simulink model "SanazMotie"  (R2021a)
settings: Solver=VariableStepAuto  StartTime=0.0  StopTime=200  RelTol=1e-3
libraries: pid_lib x7
settings Model: Creator=Sanaz  LastModifiedBy=Sanaz

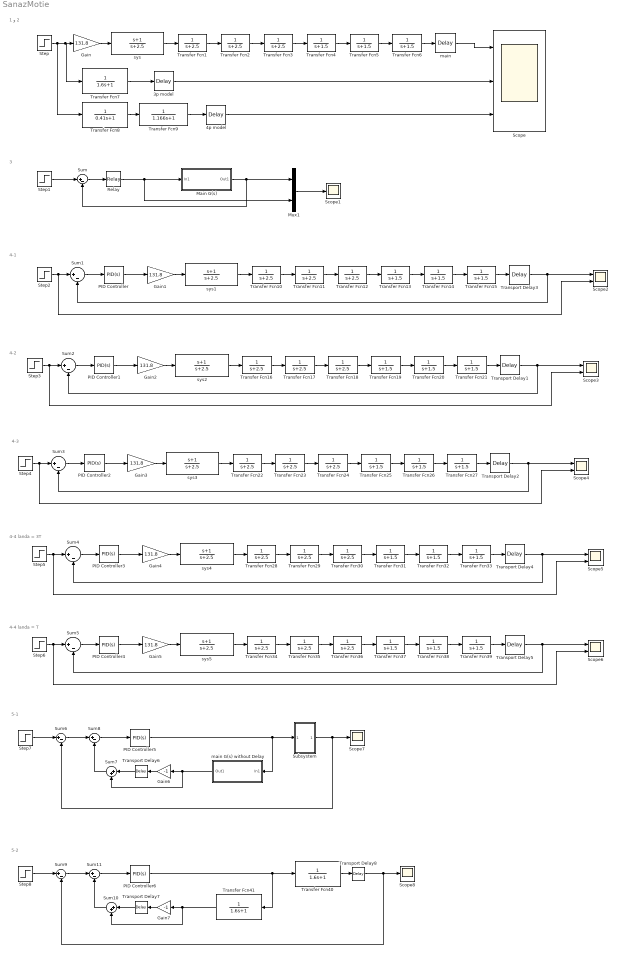
== system SanazMotie ==
  note: 5-1
  note: 3
  note: 4-1
  note: 1 و 2
  note: 4-2
  note: 4-3
  note: 4-4 landa = 3T
  note: 4-4 landa = T
  note: 5-2
  3p model : TransportDelay  DelayTime=3.7
  4p model : TransportDelay  DelayTime=3.7
  Gain{,1..5} (6 alike) : Gain  Gain=131.8
  Gain6 : Gain  Gain=-1
  Gain7 : Gain  Gain=-1
  Main G(s) : Subsystem
  Mux1 : Mux  Inputs=2
  PID Controller : pid_lib/PID Controller  Controller=PID  Form=Parallel  TimeDomain=Continuous-time  UseExternalTs=off  SampleTime=-1  IntegratorMethod=Forward Euler  FilterMethod=Forward Euler  ControllerParametersSource=internal  P=0.4  I=0.1  D=0  UseFilter=on  N=10  TunerSelectOption=Transfer Function Based (PID Tuner App)  InitialConditionSource=internal  InitialConditionForIntegrator=0  InitialConditionForFilter=0  DifferentiatorICPrevScaledInput=0  ExternalReset=none  TrackingMode=off  Kt=1  LimitOutput=off  SatLimitsSource=internal  UpperSaturationLimit=inf  LowerSaturationLimit=-inf  LinearizeAsGain=on  AntiWindupMode=none  Kb=1  POutMin=[]  POutMax=[]  IOutMin=[]  IOutMax=[]  DOutMin=[]  DOutMax=[]  NOutMin=[]  NOutMax=[]  SumOutMin=[]  SumOutMax=[]  SaturationOutMin=[]  SaturationOutMax=[]  PParamMin=[]  PParamMax=[]  IParamMin=[]  IParamMax=[]  DParamMin=[]  DParamMax=[]  NParamMin=[]  NParamMax=[]  KbParamMin=[]  KbParamMax=[]  KtParamMin=[]  KtParamMax=[]  KbOutMin=[]  KbOutMax=[]  KtOutMin=[]  KtOutMax=[]  IntegratorOutMin=[]  IntegratorOutMax=[]  FilterOutMin=[]  FilterOutMax=[]  SumI1OutMin=[]  SumI1OutMax=[]  SumI2OutMin=[]  SumI2OutMax=[]  SumI3OutMin=[]  SumI3OutMax=[]  SumI4OutMin=[]  SumI4OutMax=[]  SumDOutMin=[]  SumDOutMax=[]  DifferentiatorOutMin=[]  DifferentiatorOutMax=[]  FilterDiffOutCoefMin=[]  FilterDiffOutCoefMax=[]  ReciprocalOutMin=[]  ReciprocalOutMax=[]  SumDenOutMin=[]  SumDenOutMax=[]  SumNumOutMin=[]  SumNumOutMax=[]  DivideOutMin=[]  DivideOutMax=[]  UdiffTsProdOutMin=[]  UdiffTsProdOutMax=[]  NTsProdOutMin=[]  NTsProdOutMax=[]  UintegralTsProdOutMin=[]  UintegralTsProdOutMax=[]  UngainTsProdOutMin=[]  UngainTsProdOutMax=[]  IntegratorContinuousStateAttributes=''  IntegratorStateMustResolveToSignalObject=off  IntegratorRTWStateStorageClass=Auto  FilterContinuousStateAttributes=''  FilterStateMustResolveToSignalObject=off  FilterRTWStateStorageClass=Auto  ParallelPVariant=InternalParameters  IdealPVariant=Disabled  IVariant=InternalParameters  DVariant=InternalParameters  IntegratorVariant=Continuous  SatVariant=Disabled  AWVariant=Passthrough  PCopyVariant=Disabled  TRVariant=Disabled  FdbkBlocksVariant=Forward  IdealPFdbkVariant=Disabled  SatFdbkVariant=Disabled  DerivativeFilterVariant=ContFilter  NVariant=InternalParameters  NCopyVariant=Disabled  FilterICVariant=InternalICsFilter  IntegratorICVariant=InternalICs  ExternalResetVariant=Disabled  TRSumVariant=Passthrough  SumFdbkVariant=Disabled  SumVariant=Sum_PID  TsampFilterVariant=InternalTs  TsampNgainVariant=Passthrough  TsampIntegralVariant=Passthrough  ExternalSaturationOutDataTypeStr=Inherit: Same as second input
  PID Controller1 : pid_lib/PID Controller  Controller=PID  Form=Parallel  TimeDomain=Continuous-time  UseExternalTs=off  SampleTime=-1  IntegratorMethod=Forward Euler  FilterMethod=Forward Euler  ControllerParametersSource=internal  P=0.379787801338513  I=0.153670291898543  D=-0.495653562725149  UseFilter=on  N=0.201497063469897  TunerSelectOption=Transfer Function Based (PID Tuner App)  InitialConditionSource=internal  InitialConditionForIntegrator=0  InitialConditionForFilter=0  DifferentiatorICPrevScaledInput=0  ExternalReset=none  TrackingMode=off  Kt=1  LimitOutput=off  SatLimitsSource=internal  UpperSaturationLimit=inf  LowerSaturationLimit=-inf  LinearizeAsGain=on  AntiWindupMode=none  Kb=1  POutMin=[]  POutMax=[]  IOutMin=[]  IOutMax=[]  DOutMin=[]  DOutMax=[]  NOutMin=[]  NOutMax=[]  SumOutMin=[]  SumOutMax=[]  SaturationOutMin=[]  SaturationOutMax=[]  PParamMin=[]  PParamMax=[]  IParamMin=[]  IParamMax=[]  DParamMin=[]  DParamMax=[]  NParamMin=[]  NParamMax=[]  KbParamMin=[]  KbParamMax=[]  KtParamMin=[]  KtParamMax=[]  KbOutMin=[]  KbOutMax=[]  KtOutMin=[]  KtOutMax=[]  IntegratorOutMin=[]  IntegratorOutMax=[]  FilterOutMin=[]  FilterOutMax=[]  SumI1OutMin=[]  SumI1OutMax=[]  SumI2OutMin=[]  SumI2OutMax=[]  SumI3OutMin=[]  SumI3OutMax=[]  SumI4OutMin=[]  SumI4OutMax=[]  SumDOutMin=[]  SumDOutMax=[]  DifferentiatorOutMin=[]  DifferentiatorOutMax=[]  FilterDiffOutCoefMin=[]  FilterDiffOutCoefMax=[]  ReciprocalOutMin=[]  ReciprocalOutMax=[]  SumDenOutMin=[]  SumDenOutMax=[]  SumNumOutMin=[]  SumNumOutMax=[]  DivideOutMin=[]  DivideOutMax=[]  UdiffTsProdOutMin=[]  UdiffTsProdOutMax=[]  NTsProdOutMin=[]  NTsProdOutMax=[]  UintegralTsProdOutMin=[]  UintegralTsProdOutMax=[]  UngainTsProdOutMin=[]  UngainTsProdOutMax=[]  IntegratorContinuousStateAttributes=''  IntegratorStateMustResolveToSignalObject=off  IntegratorRTWStateStorageClass=Auto  FilterContinuousStateAttributes=''  FilterStateMustResolveToSignalObject=off  FilterRTWStateStorageClass=Auto  ParallelPVariant=InternalParameters  IdealPVariant=Disabled  IVariant=InternalParameters  DVariant=InternalParameters  IntegratorVariant=Continuous  SatVariant=Disabled  AWVariant=Passthrough  PCopyVariant=Disabled  TRVariant=Disabled  FdbkBlocksVariant=Forward  IdealPFdbkVariant=Disabled  SatFdbkVariant=Disabled  DerivativeFilterVariant=ContFilter  NVariant=InternalParameters  NCopyVariant=Disabled  FilterICVariant=InternalICsFilter  IntegratorICVariant=InternalICs  ExternalResetVariant=Disabled  TRSumVariant=Passthrough  SumFdbkVariant=Disabled  SumVariant=Sum_PID  TsampFilterVariant=InternalTs  TsampNgainVariant=Passthrough  TsampIntegralVariant=Passthrough  ExternalSaturationOutDataTypeStr=Inherit: Same as second input
  PID Controller2 : pid_lib/PID Controller  Controller=PID  Form=Parallel  TimeDomain=Continuous-time  UseExternalTs=off  SampleTime=-1  IntegratorMethod=Forward Euler  FilterMethod=Forward Euler  ControllerParametersSource=internal  P=0.258  I=0.02  D=0.6  UseFilter=on  N=3  TunerSelectOption=Frequency Response Based  InitialConditionSource=internal  InitialConditionForIntegrator=0  InitialConditionForFilter=0  DifferentiatorICPrevScaledInput=0  ExternalReset=none  TrackingMode=off  Kt=1  LimitOutput=off  SatLimitsSource=internal  UpperSaturationLimit=inf  LowerSaturationLimit=-inf  LinearizeAsGain=on  AntiWindupMode=none  Kb=1  POutMin=[]  POutMax=[]  IOutMin=[]  IOutMax=[]  DOutMin=[]  DOutMax=[]  NOutMin=[]  NOutMax=[]  SumOutMin=[]  SumOutMax=[]  SaturationOutMin=[]  SaturationOutMax=[]  PParamMin=[]  PParamMax=[]  IParamMin=[]  IParamMax=[]  DParamMin=[]  DParamMax=[]  NParamMin=[]  NParamMax=[]  KbParamMin=[]  KbParamMax=[]  KtParamMin=[]  KtParamMax=[]  KbOutMin=[]  KbOutMax=[]  KtOutMin=[]  KtOutMax=[]  IntegratorOutMin=[]  IntegratorOutMax=[]  FilterOutMin=[]  FilterOutMax=[]  SumI1OutMin=[]  SumI1OutMax=[]  SumI2OutMin=[]  SumI2OutMax=[]  SumI3OutMin=[]  SumI3OutMax=[]  SumI4OutMin=[]  SumI4OutMax=[]  SumDOutMin=[]  SumDOutMax=[]  DifferentiatorOutMin=[]  DifferentiatorOutMax=[]  FilterDiffOutCoefMin=[]  FilterDiffOutCoefMax=[]  ReciprocalOutMin=[]  ReciprocalOutMax=[]  SumDenOutMin=[]  SumDenOutMax=[]  SumNumOutMin=[]  SumNumOutMax=[]  DivideOutMin=[]  DivideOutMax=[]  UdiffTsProdOutMin=[]  UdiffTsProdOutMax=[]  NTsProdOutMin=[]  NTsProdOutMax=[]  UintegralTsProdOutMin=[]  UintegralTsProdOutMax=[]  UngainTsProdOutMin=[]  UngainTsProdOutMax=[]  IntegratorContinuousStateAttributes=''  IntegratorStateMustResolveToSignalObject=off  IntegratorRTWStateStorageClass=Auto  FilterContinuousStateAttributes=''  FilterStateMustResolveToSignalObject=off  FilterRTWStateStorageClass=Auto  ParallelPVariant=InternalParameters  IdealPVariant=Disabled  IVariant=InternalParameters  DVariant=InternalParameters  IntegratorVariant=Continuous  SatVariant=Disabled  AWVariant=Passthrough  PCopyVariant=Disabled  TRVariant=Disabled  FdbkBlocksVariant=Forward  IdealPFdbkVariant=Disabled  SatFdbkVariant=Disabled  DerivativeFilterVariant=ContFilter  NVariant=InternalParameters  NCopyVariant=Disabled  FilterICVariant=InternalICsFilter  IntegratorICVariant=InternalICs  ExternalResetVariant=Disabled  TRSumVariant=Passthrough  SumFdbkVariant=Disabled  SumVariant=Sum_PID  TsampFilterVariant=InternalTs  TsampNgainVariant=Passthrough  TsampIntegralVariant=Passthrough  ExternalSaturationOutDataTypeStr=Inherit: Same as second input
  PID Controller3 : pid_lib/PID Controller  Controller=PID  Form=Parallel  TimeDomain=Continuous-time  UseExternalTs=off  SampleTime=-1  IntegratorMethod=Forward Euler  FilterMethod=Forward Euler  ControllerParametersSource=internal  P=0.517  I=0.15  D=0.44  UseFilter=on  N=3  TunerSelectOption=Frequency Response Based  InitialConditionSource=internal  InitialConditionForIntegrator=0  InitialConditionForFilter=0  DifferentiatorICPrevScaledInput=0  ExternalReset=none  TrackingMode=off  Kt=1  LimitOutput=off  SatLimitsSource=internal  UpperSaturationLimit=inf  LowerSaturationLimit=-inf  LinearizeAsGain=on  AntiWindupMode=none  Kb=1  POutMin=[]  POutMax=[]  IOutMin=[]  IOutMax=[]  DOutMin=[]  DOutMax=[]  NOutMin=[]  NOutMax=[]  SumOutMin=[]  SumOutMax=[]  SaturationOutMin=[]  SaturationOutMax=[]  PParamMin=[]  PParamMax=[]  IParamMin=[]  IParamMax=[]  DParamMin=[]  DParamMax=[]  NParamMin=[]  NParamMax=[]  KbParamMin=[]  KbParamMax=[]  KtParamMin=[]  KtParamMax=[]  KbOutMin=[]  KbOutMax=[]  KtOutMin=[]  KtOutMax=[]  IntegratorOutMin=[]  IntegratorOutMax=[]  FilterOutMin=[]  FilterOutMax=[]  SumI1OutMin=[]  SumI1OutMax=[]  SumI2OutMin=[]  SumI2OutMax=[]  SumI3OutMin=[]  SumI3OutMax=[]  SumI4OutMin=[]  SumI4OutMax=[]  SumDOutMin=[]  SumDOutMax=[]  DifferentiatorOutMin=[]  DifferentiatorOutMax=[]  FilterDiffOutCoefMin=[]  FilterDiffOutCoefMax=[]  ReciprocalOutMin=[]  ReciprocalOutMax=[]  SumDenOutMin=[]  SumDenOutMax=[]  SumNumOutMin=[]  SumNumOutMax=[]  DivideOutMin=[]  DivideOutMax=[]  UdiffTsProdOutMin=[]  UdiffTsProdOutMax=[]  NTsProdOutMin=[]  NTsProdOutMax=[]  UintegralTsProdOutMin=[]  UintegralTsProdOutMax=[]  UngainTsProdOutMin=[]  UngainTsProdOutMax=[]  IntegratorContinuousStateAttributes=''  IntegratorStateMustResolveToSignalObject=off  IntegratorRTWStateStorageClass=Auto  FilterContinuousStateAttributes=''  FilterStateMustResolveToSignalObject=off  FilterRTWStateStorageClass=Auto  ParallelPVariant=InternalParameters  IdealPVariant=Disabled  IVariant=InternalParameters  DVariant=InternalParameters  IntegratorVariant=Continuous  SatVariant=Disabled  AWVariant=Passthrough  PCopyVariant=Disabled  TRVariant=Disabled  FdbkBlocksVariant=Forward  IdealPFdbkVariant=Disabled  SatFdbkVariant=Disabled  DerivativeFilterVariant=ContFilter  NVariant=InternalParameters  NCopyVariant=Disabled  FilterICVariant=InternalICsFilter  IntegratorICVariant=InternalICs  ExternalResetVariant=Disabled  TRSumVariant=Passthrough  SumFdbkVariant=Disabled  SumVariant=Sum_PID  TsampFilterVariant=InternalTs  TsampNgainVariant=Passthrough  TsampIntegralVariant=Passthrough  ExternalSaturationOutDataTypeStr=Inherit: Same as second input
  PID Controller4 : pid_lib/PID Controller  Controller=PID  Form=Parallel  TimeDomain=Continuous-time  UseExternalTs=off  SampleTime=-1  IntegratorMethod=Forward Euler  FilterMethod=Forward Euler  ControllerParametersSource=internal  P=1.01  I=0.3  D=0.87  UseFilter=on  N=3  TunerSelectOption=Frequency Response Based  InitialConditionSource=internal  InitialConditionForIntegrator=0  InitialConditionForFilter=0  DifferentiatorICPrevScaledInput=0  ExternalReset=none  TrackingMode=off  Kt=1  LimitOutput=off  SatLimitsSource=internal  UpperSaturationLimit=inf  LowerSaturationLimit=-inf  LinearizeAsGain=on  AntiWindupMode=none  Kb=1  POutMin=[]  POutMax=[]  IOutMin=[]  IOutMax=[]  DOutMin=[]  DOutMax=[]  NOutMin=[]  NOutMax=[]  SumOutMin=[]  SumOutMax=[]  SaturationOutMin=[]  SaturationOutMax=[]  PParamMin=[]  PParamMax=[]  IParamMin=[]  IParamMax=[]  DParamMin=[]  DParamMax=[]  NParamMin=[]  NParamMax=[]  KbParamMin=[]  KbParamMax=[]  KtParamMin=[]  KtParamMax=[]  KbOutMin=[]  KbOutMax=[]  KtOutMin=[]  KtOutMax=[]  IntegratorOutMin=[]  IntegratorOutMax=[]  FilterOutMin=[]  FilterOutMax=[]  SumI1OutMin=[]  SumI1OutMax=[]  SumI2OutMin=[]  SumI2OutMax=[]  SumI3OutMin=[]  SumI3OutMax=[]  SumI4OutMin=[]  SumI4OutMax=[]  SumDOutMin=[]  SumDOutMax=[]  DifferentiatorOutMin=[]  DifferentiatorOutMax=[]  FilterDiffOutCoefMin=[]  FilterDiffOutCoefMax=[]  ReciprocalOutMin=[]  ReciprocalOutMax=[]  SumDenOutMin=[]  SumDenOutMax=[]  SumNumOutMin=[]  SumNumOutMax=[]  DivideOutMin=[]  DivideOutMax=[]  UdiffTsProdOutMin=[]  UdiffTsProdOutMax=[]  NTsProdOutMin=[]  NTsProdOutMax=[]  UintegralTsProdOutMin=[]  UintegralTsProdOutMax=[]  UngainTsProdOutMin=[]  UngainTsProdOutMax=[]  IntegratorContinuousStateAttributes=''  IntegratorStateMustResolveToSignalObject=off  IntegratorRTWStateStorageClass=Auto  FilterContinuousStateAttributes=''  FilterStateMustResolveToSignalObject=off  FilterRTWStateStorageClass=Auto  ParallelPVariant=InternalParameters  IdealPVariant=Disabled  IVariant=InternalParameters  DVariant=InternalParameters  IntegratorVariant=Continuous  SatVariant=Disabled  AWVariant=Passthrough  PCopyVariant=Disabled  TRVariant=Disabled  FdbkBlocksVariant=Forward  IdealPFdbkVariant=Disabled  SatFdbkVariant=Disabled  DerivativeFilterVariant=ContFilter  NVariant=InternalParameters  NCopyVariant=Disabled  FilterICVariant=InternalICsFilter  IntegratorICVariant=InternalICs  ExternalResetVariant=Disabled  TRSumVariant=Passthrough  SumFdbkVariant=Disabled  SumVariant=Sum_PID  TsampFilterVariant=InternalTs  TsampNgainVariant=Passthrough  TsampIntegralVariant=Passthrough  ExternalSaturationOutDataTypeStr=Inherit: Same as second input
  PID Controller5 : pid_lib/PID Controller  Controller=PID  Form=Parallel  TimeDomain=Continuous-time  UseExternalTs=off  SampleTime=-1  IntegratorMethod=Forward Euler  FilterMethod=Forward Euler  ControllerParametersSource=internal  P=0.38  I=0.15  D=-0.5  UseFilter=on  N=0.2  TunerSelectOption=Transfer Function Based (PID Tuner App)  InitialConditionSource=internal  InitialConditionForIntegrator=0  InitialConditionForFilter=0  DifferentiatorICPrevScaledInput=0  ExternalReset=none  TrackingMode=off  Kt=1  LimitOutput=off  SatLimitsSource=internal  UpperSaturationLimit=inf  LowerSaturationLimit=-inf  LinearizeAsGain=on  AntiWindupMode=none  Kb=1  POutMin=[]  POutMax=[]  IOutMin=[]  IOutMax=[]  DOutMin=[]  DOutMax=[]  NOutMin=[]  NOutMax=[]  SumOutMin=[]  SumOutMax=[]  SaturationOutMin=[]  SaturationOutMax=[]  PParamMin=[]  PParamMax=[]  IParamMin=[]  IParamMax=[]  DParamMin=[]  DParamMax=[]  NParamMin=[]  NParamMax=[]  KbParamMin=[]  KbParamMax=[]  KtParamMin=[]  KtParamMax=[]  KbOutMin=[]  KbOutMax=[]  KtOutMin=[]  KtOutMax=[]  IntegratorOutMin=[]  IntegratorOutMax=[]  FilterOutMin=[]  FilterOutMax=[]  SumI1OutMin=[]  SumI1OutMax=[]  SumI2OutMin=[]  SumI2OutMax=[]  SumI3OutMin=[]  SumI3OutMax=[]  SumI4OutMin=[]  SumI4OutMax=[]  SumDOutMin=[]  SumDOutMax=[]  DifferentiatorOutMin=[]  DifferentiatorOutMax=[]  FilterDiffOutCoefMin=[]  FilterDiffOutCoefMax=[]  ReciprocalOutMin=[]  ReciprocalOutMax=[]  SumDenOutMin=[]  SumDenOutMax=[]  SumNumOutMin=[]  SumNumOutMax=[]  DivideOutMin=[]  DivideOutMax=[]  UdiffTsProdOutMin=[]  UdiffTsProdOutMax=[]  NTsProdOutMin=[]  NTsProdOutMax=[]  UintegralTsProdOutMin=[]  UintegralTsProdOutMax=[]  UngainTsProdOutMin=[]  UngainTsProdOutMax=[]  IntegratorContinuousStateAttributes=''  IntegratorStateMustResolveToSignalObject=off  IntegratorRTWStateStorageClass=Auto  FilterContinuousStateAttributes=''  FilterStateMustResolveToSignalObject=off  FilterRTWStateStorageClass=Auto  ParallelPVariant=InternalParameters  IdealPVariant=Disabled  IVariant=InternalParameters  DVariant=InternalParameters  IntegratorVariant=Continuous  SatVariant=Disabled  AWVariant=Passthrough  PCopyVariant=Disabled  TRVariant=Disabled  FdbkBlocksVariant=Forward  IdealPFdbkVariant=Disabled  SatFdbkVariant=Disabled  DerivativeFilterVariant=ContFilter  NVariant=InternalParameters  NCopyVariant=Disabled  FilterICVariant=InternalICsFilter  IntegratorICVariant=InternalICs  ExternalResetVariant=Disabled  TRSumVariant=Passthrough  SumFdbkVariant=Disabled  SumVariant=Sum_PID  TsampFilterVariant=InternalTs  TsampNgainVariant=Passthrough  TsampIntegralVariant=Passthrough  ExternalSaturationOutDataTypeStr=Inherit: Same as second input
  PID Controller6 : pid_lib/PID Controller  Controller=PID  Form=Parallel  TimeDomain=Continuous-time  UseExternalTs=off  SampleTime=-1  IntegratorMethod=Forward Euler  FilterMethod=Forward Euler  ControllerParametersSource=internal  P=0.38  I=0.15  D=-0.5  UseFilter=on  N=0.2  TunerSelectOption=Transfer Function Based (PID Tuner App)  InitialConditionSource=internal  InitialConditionForIntegrator=0  InitialConditionForFilter=0  DifferentiatorICPrevScaledInput=0  ExternalReset=none  TrackingMode=off  Kt=1  LimitOutput=off  SatLimitsSource=internal  UpperSaturationLimit=inf  LowerSaturationLimit=-inf  LinearizeAsGain=on  AntiWindupMode=none  Kb=1  POutMin=[]  POutMax=[]  IOutMin=[]  IOutMax=[]  DOutMin=[]  DOutMax=[]  NOutMin=[]  NOutMax=[]  SumOutMin=[]  SumOutMax=[]  SaturationOutMin=[]  SaturationOutMax=[]  PParamMin=[]  PParamMax=[]  IParamMin=[]  IParamMax=[]  DParamMin=[]  DParamMax=[]  NParamMin=[]  NParamMax=[]  KbParamMin=[]  KbParamMax=[]  KtParamMin=[]  KtParamMax=[]  KbOutMin=[]  KbOutMax=[]  KtOutMin=[]  KtOutMax=[]  IntegratorOutMin=[]  IntegratorOutMax=[]  FilterOutMin=[]  FilterOutMax=[]  SumI1OutMin=[]  SumI1OutMax=[]  SumI2OutMin=[]  SumI2OutMax=[]  SumI3OutMin=[]  SumI3OutMax=[]  SumI4OutMin=[]  SumI4OutMax=[]  SumDOutMin=[]  SumDOutMax=[]  DifferentiatorOutMin=[]  DifferentiatorOutMax=[]  FilterDiffOutCoefMin=[]  FilterDiffOutCoefMax=[]  ReciprocalOutMin=[]  ReciprocalOutMax=[]  SumDenOutMin=[]  SumDenOutMax=[]  SumNumOutMin=[]  SumNumOutMax=[]  DivideOutMin=[]  DivideOutMax=[]  UdiffTsProdOutMin=[]  UdiffTsProdOutMax=[]  NTsProdOutMin=[]  NTsProdOutMax=[]  UintegralTsProdOutMin=[]  UintegralTsProdOutMax=[]  UngainTsProdOutMin=[]  UngainTsProdOutMax=[]  IntegratorContinuousStateAttributes=''  IntegratorStateMustResolveToSignalObject=off  IntegratorRTWStateStorageClass=Auto  FilterContinuousStateAttributes=''  FilterStateMustResolveToSignalObject=off  FilterRTWStateStorageClass=Auto  ParallelPVariant=InternalParameters  IdealPVariant=Disabled  IVariant=InternalParameters  DVariant=InternalParameters  IntegratorVariant=Continuous  SatVariant=Disabled  AWVariant=Passthrough  PCopyVariant=Disabled  TRVariant=Disabled  FdbkBlocksVariant=Forward  IdealPFdbkVariant=Disabled  SatFdbkVariant=Disabled  DerivativeFilterVariant=ContFilter  NVariant=InternalParameters  NCopyVariant=Disabled  FilterICVariant=InternalICsFilter  IntegratorICVariant=InternalICs  ExternalResetVariant=Disabled  TRSumVariant=Passthrough  SumFdbkVariant=Disabled  SumVariant=Sum_PID  TsampFilterVariant=InternalTs  TsampNgainVariant=Passthrough  TsampIntegralVariant=Passthrough  ExternalSaturationOutDataTypeStr=Inherit: Same as second input
  Relay : Relay  OnOutputValue=5  OffOutputValue=-5
  Scope : Scope  NumInputPorts=3
  Scope1 : Scope
  Scope{2..6} (5 alike) : Scope  NumInputPorts=2
  Scope7 : Scope
  Scope8 : Scope
  Step{,1,7..8} (4 alike) : Step  Time=0  SampleTime=0
  Step{2..6} (5 alike) : Step  SampleTime=0
  Subsystem : Subsystem
  Sum{,1..6,8..9,11} (10 alike) : Sum  Inputs=|+-
  Sum10 : Sum  Inputs=|++
  Sum7 : Sum  Inputs=|++
  Transfer Fcn{1..3,10..12,16..18,22..24,28..30,34..36} (18 alike) : TransferFcn  Denominator=[1 2.5]
  Transfer Fcn{4..6,13..15,19..21,25..27,31..33,37..39} (18 alike) : TransferFcn  Denominator=[1 1.5]
  Transfer Fcn40 : TransferFcn  Denominator=[1.6 1]
  Transfer Fcn41 : TransferFcn  Denominator=[1.6 1]
  Transfer Fcn7 : TransferFcn  Denominator=[1.6 1]
  Transfer Fcn8 : TransferFcn  Denominator=[0.41 1]
  Transfer Fcn9 : TransferFcn  Denominator=[1.166 1]
  Transport Delay{1..5} (5 alike) : TransportDelay  DelayTime=2.5
  Transport Delay6 : TransportDelay  DelayTime=3.7
  Transport Delay7 : TransportDelay  DelayTime=3.7
  Transport Delay8 : TransportDelay  DelayTime=3.7
  main : TransportDelay  DelayTime=2.5
  main G(s) without Delay : Subsystem
  sys{,1..5} (6 alike) : TransferFcn  Numerator=[1 1]  Denominator=[1 2.5]
  wires:
  main/1 -> Scope/1
  Step/1 -> Transfer Fcn8/1, Transfer Fcn7/1, Gain/1
  Transfer Fcn3/1 -> Transfer Fcn4/1
  Transfer Fcn5/1 -> Transfer Fcn6/1
  Transfer Fcn2/1 -> Transfer Fcn3/1
  Transfer Fcn4/1 -> Transfer Fcn5/1
  Transfer Fcn6/1 -> main/1
  sys/1 -> Transfer Fcn1/1
  Transfer Fcn1/1 -> Transfer Fcn2/1
  Transfer Fcn8/1 -> Transfer Fcn9/1
  Transfer Fcn7/1 -> 3p model/1
  Transfer Fcn9/1 -> 4p model/1
  Gain/1 -> sys/1
  Step1/1 -> Sum/1
  Mux1/1 -> Scope1/1
  Relay/1 -> Mux1/2, Main G(s)/1(In1)
  Main G(s)/1(Out1) -> Sum/2, Mux1/1
  Sum/1 -> Relay/1
  Gain1/1 -> sys1/1
  Transfer Fcn10/1 -> Transfer Fcn11/1
  Transfer Fcn14/1 -> Transfer Fcn15/1
  Transfer Fcn11/1 -> Transfer Fcn12/1
  Transfer Fcn15/1 -> Transport Delay3/1
  sys1/1 -> Transfer Fcn10/1
  Transfer Fcn13/1 -> Transfer Fcn14/1
  Transfer Fcn12/1 -> Transfer Fcn13/1
  PID Controller/1 -> Gain1/1
  Step2/1 -> Scope2/2, Sum1/1
  Sum1/1 -> PID Controller/1
  Transport Delay3/1 -> Sum1/2, Scope2/1
  3p model/1 -> Scope/2
  4p model/1 -> Scope/3
  Transfer Fcn20/1 -> Transfer Fcn21/1
  Transfer Fcn18/1 -> Transfer Fcn19/1
  Transfer Fcn19/1 -> Transfer Fcn20/1
  Step3/1 -> Scope3/2, Sum2/1
  sys2/1 -> Transfer Fcn16/1
  PID Controller1/1 -> Gain2/1
  Transfer Fcn16/1 -> Transfer Fcn17/1
  Sum2/1 -> PID Controller1/1
  Transport Delay1/1 -> Sum2/2, Scope3/1
  Gain2/1 -> sys2/1
  Transfer Fcn17/1 -> Transfer Fcn18/1
  Transfer Fcn21/1 -> Transport Delay1/1
  Transport Delay2/1 -> Sum3/2, Scope4/1
  Transfer Fcn23/1 -> Transfer Fcn24/1
  Transfer Fcn27/1 -> Transport Delay2/1
  Gain3/1 -> sys3/1
  Transfer Fcn22/1 -> Transfer Fcn23/1
  Sum3/1 -> PID Controller2/1
  Step4/1 -> Scope4/2, Sum3/1
  Transfer Fcn25/1 -> Transfer Fcn26/1
  PID Controller2/1 -> Gain3/1
  Transfer Fcn24/1 -> Transfer Fcn25/1
  sys3/1 -> Transfer Fcn22/1
  Transfer Fcn26/1 -> Transfer Fcn27/1
  Transport Delay4/1 -> Sum4/2, Scope5/1
  Transfer Fcn29/1 -> Transfer Fcn30/1
  Transfer Fcn33/1 -> Transport Delay4/1
  Gain4/1 -> sys4/1
  Transfer Fcn28/1 -> Transfer Fcn29/1
  Sum4/1 -> PID Controller3/1
  Step5/1 -> Scope5/2, Sum4/1
  Transfer Fcn31/1 -> Transfer Fcn32/1
  PID Controller3/1 -> Gain4/1
  Transfer Fcn30/1 -> Transfer Fcn31/1
  sys4/1 -> Transfer Fcn28/1
  Transfer Fcn32/1 -> Transfer Fcn33/1
  PID Controller4/1 -> Gain5/1
  sys5/1 -> Transfer Fcn34/1
  Transfer Fcn38/1 -> Transfer Fcn39/1
  Transfer Fcn36/1 -> Transfer Fcn37/1
  Transfer Fcn39/1 -> Transport Delay5/1
  Sum5/1 -> PID Controller4/1
  Transfer Fcn37/1 -> Transfer Fcn38/1
  Transfer Fcn35/1 -> Transfer Fcn36/1
  Gain5/1 -> sys5/1
  Step6/1 -> Scope6/2, Sum5/1
  Transfer Fcn34/1 -> Transfer Fcn35/1
  Transport Delay5/1 -> Sum5/2, Scope6/1
  Sum7/1 -> Sum8/2
  Sum6/1 -> Sum8/1
  Subsystem/1(Out1) -> Scope7/1, Sum6/2
  Gain6/1 -> Transport Delay6/1
  Transport Delay6/1 -> Sum7/1
  main G(s) without Delay/1(Out1) -> Sum7/2, Gain6/1
  Step7/1 -> Sum6/1
  Sum8/1 -> PID Controller5/1
  PID Controller5/1 -> Subsystem/1(In1), main G(s) without Delay/1(In1)
  Sum11/1 -> PID Controller6/1
  Transfer Fcn40/1 -> Transport Delay8/1
  PID Controller6/1 -> Transfer Fcn41/1, Transfer Fcn40/1
  Step8/1 -> Sum9/1
  Gain7/1 -> Transport Delay7/1
  Transfer Fcn41/1 -> Sum10/2, Gain7/1
  Transport Delay7/1 -> Sum10/1
  Sum10/1 -> Sum11/2
  Sum9/1 -> Sum11/1
  Transport Delay8/1 -> Scope8/1, Sum9/2

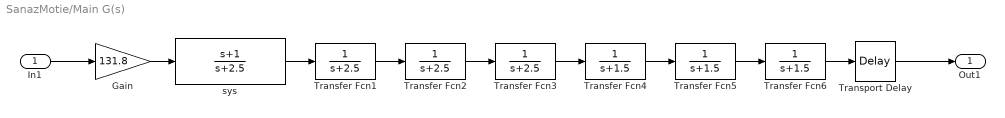
== system SanazMotie/Main G(s) ==
  In1 : Inport
  Gain : Gain  Gain=131.8
  Transfer Fcn1 : TransferFcn  Denominator=[1 2.5]
  Transfer Fcn2 : TransferFcn  Denominator=[1 2.5]
  Transfer Fcn3 : TransferFcn  Denominator=[1 2.5]
  Transfer Fcn4 : TransferFcn  Denominator=[1 1.5]
  Transfer Fcn5 : TransferFcn  Denominator=[1 1.5]
  Transfer Fcn6 : TransferFcn  Denominator=[1 1.5]
  Transport Delay : TransportDelay  DelayTime=2.5
  sys : TransferFcn  Numerator=[1 1]  Denominator=[1 2.5]
  Out1 : Outport
  wires:
  Transport Delay/1 -> Out1/1
  Transfer Fcn5/1 -> Transfer Fcn6/1
  Transfer Fcn1/1 -> Transfer Fcn2/1
  Gain/1 -> sys/1
  Transfer Fcn3/1 -> Transfer Fcn4/1
  Transfer Fcn6/1 -> Transport Delay/1
  Transfer Fcn2/1 -> Transfer Fcn3/1
  sys/1 -> Transfer Fcn1/1
  Transfer Fcn4/1 -> Transfer Fcn5/1
  In1/1 -> Gain/1

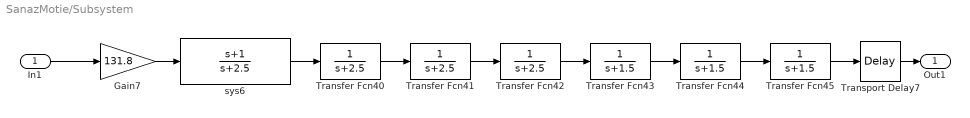
== system SanazMotie/Subsystem ==
  In1 : Inport
  Gain7 : Gain  Gain=131.8
  Transfer Fcn40 : TransferFcn  Denominator=[1 2.5]
  Transfer Fcn41 : TransferFcn  Denominator=[1 2.5]
  Transfer Fcn42 : TransferFcn  Denominator=[1 2.5]
  Transfer Fcn43 : TransferFcn  Denominator=[1 1.5]
  Transfer Fcn44 : TransferFcn  Denominator=[1 1.5]
  Transfer Fcn45 : TransferFcn  Denominator=[1 1.5]
  Transport Delay7 : TransportDelay  DelayTime=2.5
  sys6 : TransferFcn  Numerator=[1 1]  Denominator=[1 2.5]
  Out1 : Outport
  wires:
  Gain7/1 -> sys6/1
  Transfer Fcn43/1 -> Transfer Fcn44/1
  sys6/1 -> Transfer Fcn40/1
  Transfer Fcn45/1 -> Transport Delay7/1
  Transfer Fcn41/1 -> Transfer Fcn42/1
  Transfer Fcn40/1 -> Transfer Fcn41/1
  Transfer Fcn42/1 -> Transfer Fcn43/1
  Transfer Fcn44/1 -> Transfer Fcn45/1
  In1/1 -> Gain7/1
  Transport Delay7/1 -> Out1/1

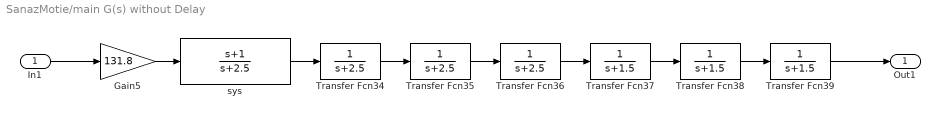
== system SanazMotie/main G(s) without Delay ==
  In1 : Inport
  Gain5 : Gain  Gain=131.8
  Transfer Fcn34 : TransferFcn  Denominator=[1 2.5]
  Transfer Fcn35 : TransferFcn  Denominator=[1 2.5]
  Transfer Fcn36 : TransferFcn  Denominator=[1 2.5]
  Transfer Fcn37 : TransferFcn  Denominator=[1 1.5]
  Transfer Fcn38 : TransferFcn  Denominator=[1 1.5]
  Transfer Fcn39 : TransferFcn  Denominator=[1 1.5]
  sys : TransferFcn  Numerator=[1 1]  Denominator=[1 2.5]
  Out1 : Outport
  wires:
  Transfer Fcn35/1 -> Transfer Fcn36/1
  Transfer Fcn37/1 -> Transfer Fcn38/1
  Gain5/1 -> sys/1
  In1/1 -> Gain5/1
  sys/1 -> Transfer Fcn34/1
  Transfer Fcn36/1 -> Transfer Fcn37/1
  Transfer Fcn38/1 -> Transfer Fcn39/1
  Transfer Fcn34/1 -> Transfer Fcn35/1
  Transfer Fcn39/1 -> Out1/1
